simulink library "tpm"  (R2021b)
settings: Solver=VariableStepAuto  StartTime=0.0  StopTime=10.0  RelTol=1e-3
undefined symbols (not defined in the file or in its folder): ENUM_AN_LF, ENUM_AN_LR, ENUM_AN_RF, ENUM_AN_RR, ENUM_POWERSTA_OFF, ENUM_POWERSTA_OFFA, ENUM_POWERSTA_OFFC, ENUM_POWERSTA_ON, ENUM_POWERSTA_READY, ENUM_POWERSTA_STANDBY, ENUM_PWRSTASW_OFF, ENUM_PWRSTASW_OFFA, ENUM_PWRSTASW_OFFCHVCHRG, ENUM_PWRSTASW_STANDBY, KTPM_Delay_raw8, KTPM_WhlRotDir_enum_ovrdflg, KTPM_WhlRotDir_enum_ovrdval, TRUE, ZERO_FLOAT, ZERO_INT
libraries: simulink x58, hcu_lib x25, $bdroot x18
(part 1 of 8)
settings Model: Creator=FVT22063  LastModifiedBy=FVT22063

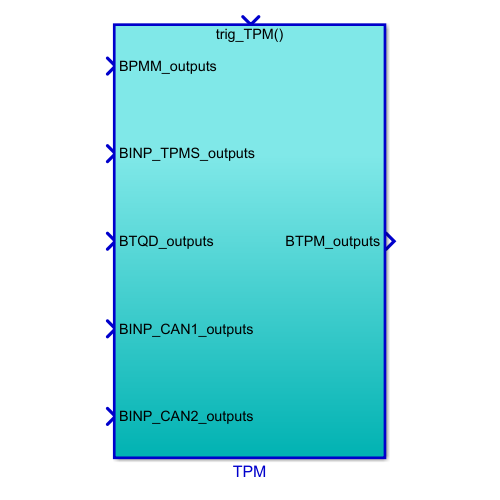
[thumbnail: Simulink's stored preview of the top-level diagram]
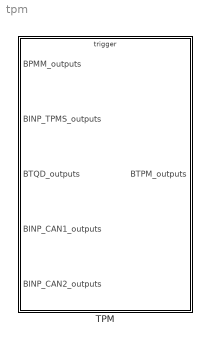
== system tpm ==
  TPM : Subsystem  TreatAsAtomicUnit=on
      settings: RTWSystemCode=Nonreusable function  RTWFcnNameOpts=Use subsystem name  RTWFileNameOpts=Use subsystem name

== system tpm/TPM ==
  note: VINP
  BPMM_outputs : Inport  OutDataTypeStr=Bus: BPMM_outputs
  BINP_TPMS_outputs : Inport  Port=2  OutDataTypeStr=Bus: BINP_TPMS_outputs
  BTQD_outputs : Inport  Port=3  OutDataTypeStr=Bus: BTQD_outputs
  BINP_CAN1_outputs : Inport  Port=4  OutDataTypeStr=Bus: BINP_CAN1_outputs
  BINP_CAN2_outputs : Inport  Port=5  OutDataTypeStr=Bus: BINP_CAN2_outputs
  trig_TPM : TriggerPort  TriggerType=function-call  VariantControl=(inherit)
  Bus Creator : BusCreator  Inputs=108  OutDataTypeStr=Bus: BTPM_outputs  NonVirtualBus=on
  Bus Selector : BusSelector  OutputSignals=VPMM_PowerSta_enum
  Bus Selector1 : BusSelector  OutputSignals=VINP_TPMSDataIn_flg,VINP_TPMSID_raw,VINP_TPMSPressure_raw,VINP_TPMSTemp_raw,VINP_TPMSFAT_flg,VINP_TPMSBattLow_flg,VINP_TPMSStorge_flg,VINP_LFID_raw,VINP_RFID_raw,VINP_LRID_raw,VINP_RRID_raw,VINP_ChkStorge_flg,VINP_ChkLFID_raw,VINP_ChkRFID_raw,VINP_ChkLRID_raw,VINP_ChkRRID_raw,VINP_FlashLFSensorFail_flg,VINP_FlashRFSensorFail_flg,VINP_FlashLRSensorFail_flg,VINP_FlashRRSensorFail_flg,VINP_FlashLFWheelPSW_raw8,VINP_FlashRFWheelPSW_raw8,VINP_FlashLRWheelPSW_raw8,VINP_FlashRRWheelPSW_raw8,VINP_FlashLFPindi_enum,VINP_FlashRFPindi_enum,VINP_FlashLRPindi_enum,VINP_FlashRRPindi_enum,VINP_FlashLFP20_raw8,VINP_FlashRFP20_raw8,VINP_FlashLRP20_raw8,VINP_FlashRRP20_raw8,VINP_FlashLFWheelPress_raw8,VINP_FlashRFWheelPress_raw8,VINP_FlashLRWheelPress_raw8,VINP_FlashRRWheelPress_raw8,VINP_FlashLFWheelTemp_C,VINP_FlashRFWheelTemp_C,VINP_FlashLRWheelTemp_C,VINP_FlashRRWheelTemp_C,VINP_FlashunlearnSfali_flg,VINP_S1ID_raw,VINP_S2ID_raw,VINP_S3ID_raw,VINP_S4ID_raw,VINP_Prepresstemptrust_flg
  Bus Selector2 : BusSelector  OutputSignals=VTQD_GearActualPosn_enum
  Bus Selector3 : BusSelector  OutputSignals=VINP_FASpeed_kph
  Bus Selector4 : BusSelector  OutputSignals=VINP_TPMSResButt_flg,VINP_TPMSCaliButt_flg,VINP_CANMsgValidIVI2_flg
  Data Type Conversion{,1..7} (8 alike) : DataTypeConversion  OutDataTypeStr=uint8
  Data Type Conversion{8..11} (4 alike) : DataTypeConversion  OutDataTypeStr=boolean
  Ground{,1..11} (12 alike) : Ground
  TPMS : Subsystem
  BTPM_outputs : Outport  OutDataTypeStr=Bus: BTPM_outputs
  wires:
  BPMM_outputs/1 -> Bus Selector/1
  BINP_TPMS_outputs/1 -> Bus Selector1/1
  BTQD_outputs/1 -> Bus Selector2/1
  BINP_CAN1_outputs/1 -> Bus Selector3/1
  BINP_CAN2_outputs/1 -> Bus Selector4/1
  Bus Creator/1 -> BTPM_outputs/1  "BTPM_outputs"
  Bus Selector/1 -> TPMS/1(VPMM_PowerSta_enum)  "<VPMM_PowerSta_enum>"
  Bus Selector1/1 -> TPMS/2(VINP_DATAin_flg)  "<VINP_TPMSDataIn_flg>"
  Bus Selector1/2 -> TPMS/3(VINP_IDin_raw32)  "<VINP_TPMSID_raw>"
  Bus Selector1/3 -> TPMS/4(VINP_Pin_raw8)  "<VINP_TPMSPressure_raw>"
  Bus Selector1/4 -> TPMS/5(VINP_Tin_raw8)  "<VINP_TPMSTemp_raw>"
  Bus Selector1/5 -> TPMS/6(VINP_FAT_flg)  "<VINP_TPMSFAT_flg>"
  Bus Selector1/6 -> TPMS/7(VINP_BatteryLow_flg)  "<VINP_TPMSBattLow_flg>"
  Bus Selector1/7 -> TPMS/8(VINP_TPMSStorge_flg)  "<VINP_TPMSStorge_flg>"
  Bus Selector1/8 -> TPMS/9(VINP_LFID_raw)  "<VINP_LFID_raw>"
  Bus Selector1/9 -> TPMS/10(VINP_RFID_raw)  "<VINP_RFID_raw>"
  Bus Selector1/10 -> TPMS/11(VINP_LRID_raw)  "<VINP_LRID_raw>"
  Bus Selector1/11 -> TPMS/12(VINP_RRID_raw)  "<VINP_RRID_raw>"
  Bus Selector1/12 -> TPMS/13(VINP_ChkStorge_flg)  "<VINP_ChkStorge_flg>"
  Bus Selector1/13 -> TPMS/14(VINP_ChkLFID_raw)  "<VINP_ChkLFID_raw>"
  Bus Selector1/14 -> TPMS/15(VINP_ChkRFID_raw)  "<VINP_ChkRFID_raw>"
  Bus Selector1/15 -> TPMS/16(VINP_ChkLRID_raw)  "<VINP_ChkLRID_raw>"
  Bus Selector1/16 -> TPMS/17(VINP_ChkRRID_raw)  "<VINP_ChkRRID_raw>"
  TPMS/14(VTPM_RFSensorFail_flg) -> Bus Creator/14
  TPMS/13(VTPM_LFSensorFail_flg) -> Bus Creator/13
  TPMS/15(VTPM_LRSensorFail_flg) -> Bus Creator/15
  TPMS/12(VTPM_RRWheelTemp_C) -> Bus Creator/12
  TPMS/16(VTPM_RRSensorFail_flg) -> Bus Creator/16
  TPMS/11("VTPM_LRWheelTemp_C ") -> Bus Creator/11
  TPMS/17(VTPM_LFWheelDebug_flg) -> Bus Creator/17
  TPMS/10("VTPM_RFWheelTemp_C ") -> Bus Creator/10
  TPMS/18(VTPM_LRWheelDebug_flg) -> Bus Creator/18
  TPMS/9("VTPM_LFWheelTemp_C ") -> Bus Creator/9
  TPMS/19(VTPM_RFWheelDebug_flg) -> Bus Creator/19
  TPMS/8(VTPM_RRWheelPress_raw8) -> Bus Creator/8
  TPMS/20(VTPM_RRWheelDebug_flg) -> Bus Creator/20
  TPMS/7(VTPM_LRWheelPress_raw8) -> Bus Creator/7
  TPMS/21(VTPM_TPMSResButtAllow_flg) -> Bus Creator/21
  TPMS/6(VTPM_RFWheelPress_raw8) -> Bus Creator/6
  TPMS/22(VTPM_TPMSCaliButtAllow_flg) -> Bus Creator/22
  TPMS/5(VTPM_LFWheelPress_raw8) -> Bus Creator/5
  TPMS/23(VTPM_LFPressIndi_enum) -> Bus Creator/23
  TPMS/4("VTPM_RRBatWarn_flg ") -> Bus Creator/4
  TPMS/24(VTPM_RFPressIndi_enum) -> Bus Creator/24
  TPMS/3("VTPM_LRBatWarn_flg ") -> Bus Creator/3
  TPMS/25(VTPM_LRPressIndi_enum) -> Bus Creator/25
  TPMS/2("VTPM_RFBatWarn_flg ") -> Bus Creator/2
  TPMS/26(VTPM_RRPressIndi_enum) -> Bus Creator/26
  TPMS/1("VTPM_LFBatWarn_flg ") -> Bus Creator/1
  TPMS/27("VTPM_TPMSWarnIndi_enum ") -> Bus Creator/27
  TPMS/28(VTPM_LFWheelTmpIndi_flg) -> Bus Creator/28
  TPMS/29(VTPM_RFWheelTmpIndi_flg) -> Bus Creator/29
  TPMS/30(VTPM_LRWheelTmpIndi_flg) -> Bus Creator/30
  TPMS/31(VTPM_RRWheelTmpIndi_flg) -> Bus Creator/31
  TPMS/32(VTPM_LFWheelPSW_raw8) -> Bus Creator/32
  TPMS/33(VTPM_LRWheelPSW_raw8) -> Bus Creator/33
  TPMS/34(VTPM_RFWheelPSW_raw8) -> Bus Creator/34
  TPMS/35(VTPM_RRWheelPSW_raw8) -> Bus Creator/35
  TPMS/36(VTPM_LFS1_cnt) -> Bus Creator/36
  TPMS/37(VTPM_RFS1_cnt) -> Bus Creator/37
  TPMS/38(VTPM_RRS1_cnt) -> Bus Creator/38
  TPMS/39(VTPM_LRS1_cnt) -> Bus Creator/39
  TPMS/40(VTPM_LFS2_cnt) -> Bus Creator/40
  TPMS/41(VTPM_RFS2_cnt) -> Bus Creator/41
  TPMS/42(VTPM_RRS2_cnt) -> Bus Creator/42
  TPMS/43(VTPM_LRS2_cnt) -> Bus Creator/43
  TPMS/44(VTPM_LFS3_cnt) -> Bus Creator/44
  TPMS/45(VTPM_RFS3_cnt) -> Bus Creator/45
  TPMS/46(VTPM_RRS3_cnt) -> Bus Creator/46
  TPMS/47(VTPM_LRS3_cnt) -> Bus Creator/47
  TPMS/48(VTPM_LFS4_cnt) -> Bus Creator/48
  TPMS/49(VTPM_RFS4_cnt) -> Bus Creator/49
  TPMS/50(VTPM_RRS4_cnt) -> Bus Creator/50
  TPMS/51(VTPM_LRS4_cnt) -> Bus Creator/51
  TPMS/52(VTPM_CWheelTips_enum) -> Bus Creator/52
  TPMS/53(VTPM_AutoLTips_enum) -> Bus Creator/53
  TPMS/54(VTPM_LFSensorMode_flg) -> Bus Creator/54
  TPMS/55(VTPM_RFSensorMode_flg) -> Bus Creator/55
  TPMS/56(VTPM_LRSensorMode_flg) -> Bus Creator/56
  TPMS/57(VTPM_RRSensorMode_flg) -> Bus Creator/57
  TPMS/58(VTPM_S1ID_raw32) -> Bus Creator/58
  TPMS/59(VTPM_S2ID_raw32) -> Bus Creator/59
  TPMS/60(VTPM_S3ID_raw32) -> Bus Creator/60
  TPMS/61(VTPM_S4ID_raw32) -> Bus Creator/61
  TPMS/62(VTPM_S1L_enum) -> Bus Creator/62
  TPMS/63(VTPM_S2L_enum) -> Bus Creator/63
  TPMS/64(VTPM_S3L_enum) -> Bus Creator/64
  TPMS/65(VTPM_S4L_enum) -> Bus Creator/65
  TPMS/66(VTPM_ALFin_flg) -> Bus Creator/66
  TPMS/67(VTPM_IDLOCK_flg) -> Bus Creator/67
  TPMS/68(VTPM_LFP20_raw8) -> Bus Creator/68
  TPMS/69(VTPM_RFP20_raw8) -> Bus Creator/69
  TPMS/70(VTPM_LRP20_raw8) -> Bus Creator/70
  TPMS/71(VTPM_RRP20_raw8) -> Bus Creator/71
  TPMS/72(VTPM_FAT_flg) -> Bus Creator/72
  TPMS/73(VTPM_IDin_raw32) -> Bus Creator/73
  TPMS/74(VTPM_S1WheelDebugALTU_pct) -> Bus Creator/74
  TPMS/75(VTPM_S2WheelDebugALTU_pct) -> Bus Creator/75
  TPMS/76(VTPM_S3WheelDebugALTU_pct) -> Bus Creator/76
  TPMS/77(VTPM_S4WheelDebugALTU_pct) -> Bus Creator/77
  TPMS/78(VTPM_ID1messageALTU_raw8) -> Bus Creator/78
  TPMS/79(VTPM_ID2messageALTU_raw8) -> Bus Creator/79
  TPMS/80(VTPM_ID3messageALTU_raw8) -> Bus Creator/80
  TPMS/81(VTPM_ID4messageALTU_raw8) -> Bus Creator/81
  TPMS/82(VTPM_Chkfin_flg) -> Bus Creator/82
  TPMS/83(VTPM_SetIDLoc_flg) -> Bus Creator/83
  TPMS/84(VTPM_TPMSStorge_flg) -> Bus Creator/84
  TPMS/85(VTPM_ChkStorge_flg) -> Bus Creator/85
  TPMS/86(VTPM_TPMSResButt_flg) -> Bus Creator/86
  TPMS/87(VTPM_LFPindi_enum) -> Bus Creator/87
  TPMS/88(VTPM_RFPind_enum) -> Bus Creator/88
  TPMS/89(VTPM_LRPindi_enum) -> Bus Creator/89
  TPMS/90(VTPM_RRPindi_enum) -> Bus Creator/90
  TPMS/91(VTPM_WriteChkLFID_raw) -> Bus Creator/91
  TPMS/92(VTPM_WriteChkRFID_raw) -> Bus Creator/92
  TPMS/93(VTPM_WriteChkLRID_raw) -> Bus Creator/93
  TPMS/94(VTPM_WriteChkRRID_raw) -> Bus Creator/94
  TPMS/95(VTPM_WriteChkfinLFID_raw) -> Bus Creator/95
  TPMS/96(VTPM_WriteChkfinRFID_raw) -> Bus Creator/96
  TPMS/97(VTPM_WriteChkfinLRID_raw) -> Bus Creator/97
  TPMS/98(VTPM_WriteChkfinRRID_raw) -> Bus Creator/98
  TPMS/99(VTPM_Flashchkdatavalid_enum) -> Bus Creator/99
  TPMS/100(VTPM_Flashdatavalid_enum) -> Bus Creator/100
  TPMS/101(VTPM_unlearnSfali_flg) -> Bus Creator/101
  Bus Selector1/17 -> TPMS/18(VINP_FlashLFSensorFail_flg)  "<VINP_FlashLFSensorFail_flg>"
  Bus Selector1/18 -> TPMS/19(VINP_FlashRFSensorFail_flg)  "<VINP_FlashRFSensorFail_flg>"
  Bus Selector1/19 -> TPMS/20(VINP_FlashLRSensorFail_flg)  "<VINP_FlashLRSensorFail_flg>"
  Bus Selector1/20 -> TPMS/21(VINP_FlashRRSensorFail_flg)  "<VINP_FlashRRSensorFail_flg>"
  Bus Selector1/21 -> TPMS/22(VINP_FlashLFWheelPSW_raw8)  "<VINP_FlashLFWheelPSW_raw8>"
  Bus Selector1/22 -> TPMS/23(VINP_FlashRFWheelPSW_raw8)  "<VINP_FlashRFWheelPSW_raw8>"
  Bus Selector1/23 -> TPMS/24(VINP_FlashLRWheelPSW_raw8)  "<VINP_FlashLRWheelPSW_raw8>"
  Bus Selector1/24 -> TPMS/25(VINP_FlashRRWheelPSW_raw8)  "<VINP_FlashRRWheelPSW_raw8>"
  Bus Selector1/25 -> TPMS/26(VINP_FlashLFPindi_enum)  "<VINP_FlashLFPindi_enum>"
  Bus Selector1/26 -> TPMS/27(VINP_FlashRFPindi_enum)  "<VINP_FlashRFPindi_enum>"
  Bus Selector1/27 -> TPMS/28(VINP_FlashLRPindi_enum)  "<VINP_FlashLRPindi_enum>"
  Bus Selector1/28 -> TPMS/29(VINP_FlashRRPindi_enum)  "<VINP_FlashRRPindi_enum>"
  Bus Selector1/29 -> TPMS/30(VINP_FlashLFP20_raw8)  "<VINP_FlashLFP20_raw8>"
  Bus Selector1/30 -> TPMS/31(VINP_FlashRFP20_raw8)  "<VINP_FlashRFP20_raw8>"
  Bus Selector1/31 -> TPMS/32(VINP_FlashLRP20_raw8)  "<VINP_FlashLRP20_raw8>"
  Bus Selector1/32 -> TPMS/33(VINP_FlashRRP20_raw8)  "<VINP_FlashRRP20_raw8>"
  Bus Selector1/33 -> TPMS/34(VINP_FlashLFWheelPress_raw8)  "<VINP_FlashLFWheelPress_raw8>"
  Bus Selector1/34 -> TPMS/35(VINP_FlashRFWheelPress_raw8)  "<VINP_FlashRFWheelPress_raw8>"
  Bus Selector1/35 -> TPMS/36(VINP_FlashLRFWheelPress_raw8)  "<VINP_FlashLRWheelPress_raw8>"
  Bus Selector1/36 -> TPMS/37(VINP_FlashRRWheelPress_raw8)  "<VINP_FlashRRWheelPress_raw8>"
  Bus Selector1/37 -> TPMS/38(VINP_FlashLFWheelTemp_C)  "<VINP_FlashLFWheelTemp_C>"
  Bus Selector1/38 -> TPMS/39(VINP_FlashRFWheelTemp_C)  "<VINP_FlashRFWheelTemp_C>"
  Bus Selector1/39 -> TPMS/40(VINP_FlashLRWheelTemp_C)  "<VINP_FlashLRWheelTemp_C>"
  Bus Selector1/40 -> TPMS/41(VINP_FlashRRWheelTemp_C)  "<VINP_FlashRRWheelTemp_C>"
  Bus Selector1/41 -> TPMS/42(VINP_FlashunlearnSfali_flg)  "<VINP_FlashunlearnSfali_flg>"
  Bus Selector4/1 -> TPMS/61(VINP_TPMSResButt_flg)  "<VINP_TPMSResButt_flg>"
  Bus Selector4/2 -> TPMS/62(VINP_TPMSCaliButt_flg)  "<VINP_TPMSCaliButt_flg>"
  Bus Selector4/3 -> TPMS/63(VINP_IVICANValid_flg)  "<VINP_CANMsgValidIVI2_flg>"
  Bus Selector2/1 -> TPMS/64(VTQD_GearActualPosn_enum)  "<VTQD_GearActualPosn_enum>"
  TPMS/102(VTPM_unlearnSfailvalid_enum) -> Bus Creator/102
  TPMS/103(VTPM_Prepresstempvalid_enum) -> Bus Creator/103
  Bus Selector1/42 -> TPMS/43(VINP_S1ID_raw)  "<VINP_S1ID_raw>"
  Bus Selector1/43 -> TPMS/44(VINP_S2ID_raw)  "<VINP_S2ID_raw>"
  Bus Selector1/44 -> TPMS/45(VINP_S3ID_raw)  "<VINP_S3ID_raw>"
  Bus Selector1/45 -> TPMS/46(VINP_S4ID_raw)  "<VINP_S4ID_raw>"
  TPMS/104(VTPM_FlashS1ID_raw) -> Bus Creator/104
  TPMS/105(VTPM_FlashS2ID_raw) -> Bus Creator/105
  TPMS/106(VTPM_FlashS3ID_raw) -> Bus Creator/106
  TPMS/107(VTPM_FlashS4ID_raw) -> Bus Creator/107
  TPMS/108(VTPM_FlashIDvalid_enum) -> Bus Creator/108
  Bus Selector1/46 -> TPMS/47(VINP_Prepresstemptrust_flg)  "<VINP_Prepresstemptrust_flg>"
  Bus Selector3/1 -> TPMS/60(VINP_VehSpeed_kph)  "<VINP_FASpeed_kph>"
  Ground/1 -> Data Type Conversion/1
  Ground1/1 -> Data Type Conversion1/1
  Ground2/1 -> Data Type Conversion2/1
  Ground3/1 -> Data Type Conversion3/1
  Ground4/1 -> Data Type Conversion8/1
  Ground5/1 -> Data Type Conversion9/1
  Ground6/1 -> Data Type Conversion10/1
  Ground7/1 -> Data Type Conversion11/1
  Ground8/1 -> Data Type Conversion4/1
  Ground9/1 -> Data Type Conversion5/1
  Ground10/1 -> Data Type Conversion6/1
  Ground11/1 -> Data Type Conversion7/1
  Data Type Conversion/1 -> TPMS/48(VINP_LFPulseCount_cnt)
  Data Type Conversion1/1 -> TPMS/49(VINP_RFPulseCount_cnt)
  Data Type Conversion2/1 -> TPMS/50(VINP_LRPulseCount_cnt)
  Data Type Conversion3/1 -> TPMS/51(VINP_RRPulseCount_cnt)
  Data Type Conversion4/1 -> TPMS/56(VINP_LFWhlRotDir_enum)
  Data Type Conversion5/1 -> TPMS/57(VINP_RFWhlRotDir_enum)
  Data Type Conversion6/1 -> TPMS/58(VINP_LRWhlRotDir_enum)
  Data Type Conversion7/1 -> TPMS/59(VINP_RRWhlRotDir_enum)
  Data Type Conversion8/1 -> TPMS/52(VINP_LFPulseCountV_flg)
  Data Type Conversion9/1 -> TPMS/53(VINP_RFPulseCountV_flg)
  Data Type Conversion10/1 -> TPMS/54(VINP_LRPulseCountV_flg)
  Data Type Conversion11/1 -> TPMS/55(VINP_RRPulseCountV_flg)

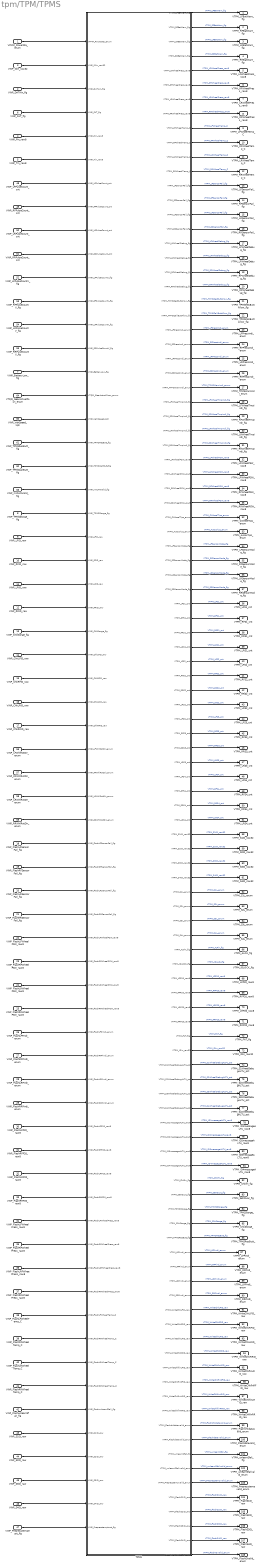
== system tpm/TPM/TPMS ==
  VPMM_PowerSta_enum : Inport
  VINP_DATAin_flg : Inport  Port=2
  VINP_IDin_raw32 : Inport  Port=3
  VINP_Pin_raw8 : Inport  Port=4
  VINP_Tin_raw8 : Inport  Port=5
  VINP_FAT_flg : Inport  Port=6
  VINP_BatteryLow_flg : Inport  Port=7
  VINP_TPMSStorge_flg : Inport  Port=8
  VINP_LFID_raw : Inport  Port=9
  VINP_RFID_raw : Inport  Port=10
  VINP_LRID_raw : Inport  Port=11
  VINP_RRID_raw : Inport  Port=12
  VINP_ChkStorge_flg : Inport  Port=13
  VINP_ChkLFID_raw : Inport  Port=14
  VINP_ChkRFID_raw : Inport  Port=15
  VINP_ChkLRID_raw : Inport  Port=16
  VINP_ChkRRID_raw : Inport  Port=17
  VINP_FlashLFSensorFail_flg : Inport  Port=18
  VINP_FlashRFSensorFail_flg : Inport  Port=19
  VINP_FlashLRSensorFail_flg : Inport  Port=20
  VINP_FlashRRSensorFail_flg : Inport  Port=21
  VINP_FlashLFWheelPSW_raw8 : Inport  Port=22
  VINP_FlashRFWheelPSW_raw8 : Inport  Port=23
  VINP_FlashLRWheelPSW_raw8 : Inport  Port=24
  VINP_FlashRRWheelPSW_raw8 : Inport  Port=25
  VINP_FlashLFPindi_enum : Inport  Port=26
  VINP_FlashRFPindi_enum : Inport  Port=27
  VINP_FlashLRPindi_enum : Inport  Port=28
  VINP_FlashRRPindi_enum : Inport  Port=29
  VINP_FlashLFP20_raw8 : Inport  Port=30
  VINP_FlashRFP20_raw8 : Inport  Port=31
  VINP_FlashLRP20_raw8 : Inport  Port=32
  VINP_FlashRRP20_raw8 : Inport  Port=33
  VINP_FlashLFWheelPress_raw8 : Inport  Port=34
  VINP_FlashRFWheelPress_raw8 : Inport  Port=35
  VINP_FlashLRFWheelPress_raw8 : Inport  Port=36
  VINP_FlashRRWheelPress_raw8 : Inport  Port=37
  VINP_FlashLFWheelTemp_C : Inport  Port=38
  VINP_FlashRFWheelTemp_C : Inport  Port=39
  VINP_FlashLRWheelTemp_C : Inport  Port=40
  VINP_FlashRRWheelTemp_C : Inport  Port=41
  VINP_FlashunlearnSfali_flg : Inport  Port=42
  VINP_S1ID_raw : Inport  Port=43
  VINP_S2ID_raw : Inport  Port=44
  VINP_S3ID_raw : Inport  Port=45
  VINP_S4ID_raw : Inport  Port=46
  VINP_Prepresstemptrust_flg : Inport  Port=47
  VINP_LFPulseCount_cnt : Inport  Port=48
  VINP_RFPulseCount_cnt : Inport  Port=49
  VINP_LRPulseCount_cnt : Inport  Port=50
  VINP_RRPulseCount_cnt : Inport  Port=51
  VINP_LFPulseCountV_flg : Inport  Port=52
  VINP_RFPulseCountV_flg : Inport  Port=53
  VINP_LRPulseCountV_flg : Inport  Port=54
  VINP_RRPulseCountV_flg : Inport  Port=55
  VINP_LFWhlRotDir_enum : Inport  Port=56
  VINP_RFWhlRotDir_enum : Inport  Port=57
  VINP_LRWhlRotDir_enum : Inport  Port=58
  VINP_RRWhlRotDir_enum : Inport  Port=59
  VINP_VehSpeed_kph : Inport  Port=60
  VINP_TPMSResButt_flg : Inport  Port=61
  VINP_TPMSCaliButt_flg : Inport  Port=62
  VINP_IVICANValid_flg : Inport  Port=63
  VTQD_GearActualPosn_enum : Inport  Port=64
  TPMS : Subsystem
  "VTPM_LFBatWarn_flg " : Outport
  "VTPM_RFBatWarn_flg " : Outport  Port=2
  "VTPM_LRBatWarn_flg " : Outport  Port=3
  "VTPM_RRBatWarn_flg " : Outport  Port=4
  VTPM_LFWheelPress_raw8 : Outport  Port=5
  VTPM_RFWheelPress_raw8 : Outport  Port=6
  VTPM_LRWheelPress_raw8 : Outport  Port=7
  VTPM_RRWheelPress_raw8 : Outport  Port=8
  "VTPM_LFWheelTemp_C " : Outport  Port=9
  "VTPM_RFWheelTemp_C " : Outport  Port=10
  "VTPM_LRWheelTemp_C " : Outport  Port=11
  VTPM_RRWheelTemp_C : Outport  Port=12
  VTPM_LFSensorFail_flg : Outport  Port=13
  VTPM_RFSensorFail_flg : Outport  Port=14
  VTPM_LRSensorFail_flg : Outport  Port=15
  VTPM_RRSensorFail_flg : Outport  Port=16
  VTPM_LFWheelDebug_flg : Outport  Port=17
  VTPM_LRWheelDebug_flg : Outport  Port=18
  VTPM_RFWheelDebug_flg : Outport  Port=19
  VTPM_RRWheelDebug_flg : Outport  Port=20
  VTPM_TPMSResButtAllow_flg : Outport  Port=21
  VTPM_TPMSCaliButtAllow_flg : Outport  Port=22
  VTPM_LFPressIndi_enum : Outport  Port=23
  VTPM_RFPressIndi_enum : Outport  Port=24
  VTPM_LRPressIndi_enum : Outport  Port=25
  VTPM_RRPressIndi_enum : Outport  Port=26
  "VTPM_TPMSWarnIndi_enum " : Outport  Port=27
  VTPM_LFWheelTmpIndi_flg : Outport  Port=28
  VTPM_RFWheelTmpIndi_flg : Outport  Port=29
  VTPM_LRWheelTmpIndi_flg : Outport  Port=30
  VTPM_RRWheelTmpIndi_flg : Outport  Port=31
  VTPM_LFWheelPSW_raw8 : Outport  Port=32
  VTPM_LRWheelPSW_raw8 : Outport  Port=33
  VTPM_RFWheelPSW_raw8 : Outport  Port=34
  VTPM_RRWheelPSW_raw8 : Outport  Port=35
  VTPM_LFS1_cnt : Outport  Port=36
  VTPM_RFS1_cnt : Outport  Port=37
  VTPM_RRS1_cnt : Outport  Port=38
  VTPM_LRS1_cnt : Outport  Port=39
  VTPM_LFS2_cnt : Outport  Port=40
  VTPM_RFS2_cnt : Outport  Port=41
  VTPM_RRS2_cnt : Outport  Port=42
  VTPM_LRS2_cnt : Outport  Port=43
  VTPM_LFS3_cnt : Outport  Port=44
  VTPM_RFS3_cnt : Outport  Port=45
  VTPM_RRS3_cnt : Outport  Port=46
  VTPM_LRS3_cnt : Outport  Port=47
  VTPM_LFS4_cnt : Outport  Port=48
  VTPM_RFS4_cnt : Outport  Port=49
  VTPM_RRS4_cnt : Outport  Port=50
  VTPM_LRS4_cnt : Outport  Port=51
  VTPM_CWheelTips_enum : Outport  Port=52
  VTPM_AutoLTips_enum : Outport  Port=53
  VTPM_LFSensorMode_flg : Outport  Port=54
  VTPM_RFSensorMode_flg : Outport  Port=55
  VTPM_LRSensorMode_flg : Outport  Port=56
  VTPM_RRSensorMode_flg : Outport  Port=57
  VTPM_S1ID_raw32 : Outport  Port=58
  VTPM_S2ID_raw32 : Outport  Port=59
  VTPM_S3ID_raw32 : Outport  Port=60
  VTPM_S4ID_raw32 : Outport  Port=61
  VTPM_S1L_enum : Outport  Port=62
  VTPM_S2L_enum : Outport  Port=63
  VTPM_S3L_enum : Outport  Port=64
  VTPM_S4L_enum : Outport  Port=65
  VTPM_ALFin_flg : Outport  Port=66
  VTPM_IDLOCK_flg : Outport  Port=67
  VTPM_LFP20_raw8 : Outport  Port=68
  VTPM_RFP20_raw8 : Outport  Port=69
  VTPM_LRP20_raw8 : Outport  Port=70
  VTPM_RRP20_raw8 : Outport  Port=71
  VTPM_FAT_flg : Outport  Port=72
  VTPM_IDin_raw32 : Outport  Port=73
  VTPM_S1WheelDebugALTU_pct : Outport  Port=74
  VTPM_S2WheelDebugALTU_pct : Outport  Port=75
  VTPM_S3WheelDebugALTU_pct : Outport  Port=76
  VTPM_S4WheelDebugALTU_pct : Outport  Port=77
  VTPM_ID1messageALTU_raw8 : Outport  Port=78
  VTPM_ID2messageALTU_raw8 : Outport  Port=79
  VTPM_ID3messageALTU_raw8 : Outport  Port=80
  VTPM_ID4messageALTU_raw8 : Outport  Port=81
  VTPM_Chkfin_flg : Outport  Port=82
  VTPM_SetIDLoc_flg : Outport  Port=83
  VTPM_TPMSStorge_flg : Outport  Port=84
  VTPM_ChkStorge_flg : Outport  Port=85
  VTPM_TPMSResButt_flg : Outport  Port=86
  VTPM_LFPindi_enum : Outport  Port=87
  VTPM_RFPind_enum : Outport  Port=88
  VTPM_LRPindi_enum : Outport  Port=89
  VTPM_RRPindi_enum : Outport  Port=90
  VTPM_WriteChkLFID_raw : Outport  Port=91
  VTPM_WriteChkRFID_raw : Outport  Port=92
  VTPM_WriteChkLRID_raw : Outport  Port=93
  VTPM_WriteChkRRID_raw : Outport  Port=94
  VTPM_WriteChkfinLFID_raw : Outport  Port=95
  VTPM_WriteChkfinRFID_raw : Outport  Port=96
  VTPM_WriteChkfinLRID_raw : Outport  Port=97
  VTPM_WriteChkfinRRID_raw : Outport  Port=98
  VTPM_Flashchkdatavalid_enum : Outport  Port=99
  VTPM_Flashdatavalid_enum : Outport  Port=100
  VTPM_unlearnSfali_flg : Outport  Port=101
  VTPM_unlearnSfailvalid_enum : Outport  Port=102
  VTPM_Prepresstempvalid_enum : Outport  Port=103
  VTPM_FlashS1ID_raw : Outport  Port=104
  VTPM_FlashS2ID_raw : Outport  Port=105
  VTPM_FlashS3ID_raw : Outport  Port=106
  VTPM_FlashS4ID_raw : Outport  Port=107
  VTPM_FlashIDvalid_enum : Outport  Port=108
  wires:
  TPMS/87(VTPM_LFPindi_enum) -> VTPM_LFPindi_enum/1  "VTPM_LFPindi_enum"
  TPMS/1("VTPM_LFBatWarn_flg ") -> "VTPM_LFBatWarn_flg "/1  "VTPM_LFBatWarn_flg"
  TPMS/2("VTPM_RFBatWarn_flg ") -> "VTPM_RFBatWarn_flg "/1  "VTPM_RFBatWarn_flg"
  TPMS/3("VTPM_LRBatWarn_flg ") -> "VTPM_LRBatWarn_flg "/1  "VTPM_LRBatWarn_flg"
  TPMS/4("VTPM_RRBatWarn_flg ") -> "VTPM_RRBatWarn_flg "/1  "VTPM_RRBatWarn_flg"
  TPMS/5(VTPM_LFWheelPress_raw8) -> VTPM_LFWheelPress_raw8/1  "VTPM_LFWheelPress_raw8"
  TPMS/6(VTPM_RFWheelPress_raw8) -> VTPM_RFWheelPress_raw8/1  "VTPM_RFWheelPress_raw8"
  TPMS/7(VTPM_LRWheelPress_raw8) -> VTPM_LRWheelPress_raw8/1  "VTPM_LRWheelPress_raw8"
  TPMS/8(VTPM_RRWheelPress_raw8) -> VTPM_RRWheelPress_raw8/1  "VTPM_RRWheelPress_raw8"
  TPMS/9("VTPM_LFWheelTemp_C ") -> "VTPM_LFWheelTemp_C "/1  "VTPM_LFWheelTemp_C"
  TPMS/10("VTPM_RFWheelTemp_C ") -> "VTPM_RFWheelTemp_C "/1  "VTPM_RFWheelTemp_C"
  TPMS/11("VTPM_LRWheelTemp_C ") -> "VTPM_LRWheelTemp_C "/1  "VTPM_LRWheelTemp_C"
  TPMS/12(VTPM_RRWheelTemp_C) -> VTPM_RRWheelTemp_C/1  "VTPM_RRWheelTemp_C"
  TPMS/13(VTPM_LFSensorFail_flg) -> VTPM_LFSensorFail_flg/1  "VTPM_LFSensorFail_flg"
  TPMS/14(VTPM_RFSensorFail_flg) -> VTPM_RFSensorFail_flg/1  "VTPM_RFSensorFail_flg"
  TPMS/15(VTPM_LRSensorFail_flg) -> VTPM_LRSensorFail_flg/1  "VTPM_LRSensorFail_flg"
  TPMS/16(VTPM_RRSensorFail_flg) -> VTPM_RRSensorFail_flg/1  "VTPM_RRSensorFail_flg"
  TPMS/17(VTPM_LFWheelDebug_flg) -> VTPM_LFWheelDebug_flg/1  "VTPM_LFWheelDebug_flg"
  TPMS/18(VTPM_LRWheelDebug_flg) -> VTPM_LRWheelDebug_flg/1  "VTPM_LRWheelDebug_flg"
  TPMS/19(VTPM_RFWheelDebug_flg) -> VTPM_RFWheelDebug_flg/1  "VTPM_RFWheelDebug_flg"
  TPMS/20(VTPM_RRWheelDebug_flg) -> VTPM_RRWheelDebug_flg/1  "VTPM_RRWheelDebug_flg"
  TPMS/21(VTPM_TPMSResButtAllow_flg) -> VTPM_TPMSResButtAllow_flg/1  "VTPM_TPMSResButtAllow_flg"
  TPMS/22(VTPM_TPMSCaliButtAllow_flg) -> VTPM_TPMSCaliButtAllow_flg/1  "VTPM_TPMSCaliButtAllow_flg"
  TPMS/23(VTPM_LFPressIndi_enum) -> VTPM_LFPressIndi_enum/1  "VTPM_LFPressIndi_enum"
  TPMS/24(VTPM_RFPressIndi_enum) -> VTPM_RFPressIndi_enum/1  "VTPM_RFPressIndi_enum"
  TPMS/25(VTPM_LRPressIndi_enum) -> VTPM_LRPressIndi_enum/1  "VTPM_LRPressIndi_enum"
  TPMS/26(VTPM_RRPressIndi_enum) -> VTPM_RRPressIndi_enum/1  "VTPM_RRPressIndi_enum"
  TPMS/27("VTPM_TPMSWarnIndi_enum ") -> "VTPM_TPMSWarnIndi_enum "/1  "VTPM_TPMSWarnIndi_enum"
  TPMS/28(VTPM_LFWheelTmpIndi_flg) -> VTPM_LFWheelTmpIndi_flg/1  "VTPM_LFWheelTmpIndi_flg"
  TPMS/29(VTPM_RFWheelTmpIndi_flg) -> VTPM_RFWheelTmpIndi_flg/1  "VTPM_RFWheelTmpIndi_flg"
  TPMS/30(VTPM_LRWheelTmpIndi_flg) -> VTPM_LRWheelTmpIndi_flg/1  "VTPM_LRWheelTmpIndi_flg"
  TPMS/31(VTPM_RRWheelTmpIndi_flg) -> VTPM_RRWheelTmpIndi_flg/1  "VTPM_RRWheelTmpIndi_flg"
  TPMS/32(VTPM_LFWheelPSW_raw8) -> VTPM_LFWheelPSW_raw8/1  "VTPM_LFWheelPSW_raw8"
  TPMS/33(VTPM_LRWheelPSW_raw8) -> VTPM_LRWheelPSW_raw8/1  "VTPM_LRWheelPSW_raw8"
  TPMS/34(VTPM_RFWheelPSW_raw8) -> VTPM_RFWheelPSW_raw8/1  "VTPM_RFWheelPSW_raw8"
  TPMS/35(VTPM_RRWheelPSW_raw8) -> VTPM_RRWheelPSW_raw8/1  "VTPM_RRWheelPSW_raw8"
  TPMS/36(VTPM_CWheelTips_enum) -> VTPM_CWheelTips_enum/1  "VTPM_CWheelTips_enum"
  TPMS/37(VTPM_AutoLTips_enum) -> VTPM_AutoLTips_enum/1  "VTPM_AutoLTips_enum"
  TPMS/38(VTPM_LFSensorMode_flg) -> VTPM_LFSensorMode_flg/1  "VTPM_LFSensorMode_flg"
  TPMS/39(VTPM_RFSensorMode_flg) -> VTPM_RFSensorMode_flg/1  "VTPM_RFSensorMode_flg"
  TPMS/40(VTPM_LRSensorMode_flg) -> VTPM_LRSensorMode_flg/1  "VTPM_LRSensorMode_flg"
  TPMS/41(VTPM_RRSensorMode_flg) -> VTPM_RRSensorMode_flg/1  "VTPM_RRSensorMode_flg"
  TPMS/42(VTPM_LFS1_cnt) -> VTPM_LFS1_cnt/1  "VTPM_LFS1_cnt"
  TPMS/43(VTPM_RFS1_cnt) -> VTPM_RFS1_cnt/1  "VTPM_RFS1_cnt"
  TPMS/44(VTPM_RRS1_cnt) -> VTPM_RRS1_cnt/1  "VTPM_RRS1_cnt"
  TPMS/45(VTPM_LRS1_cnt) -> VTPM_LRS1_cnt/1  "VTPM_LRS1_cnt"
  TPMS/46(VTPM_LFS2_cnt) -> VTPM_LFS2_cnt/1  "VTPM_LFS2_cnt"
  TPMS/47(VTPM_RFS2_cnt) -> VTPM_RFS2_cnt/1  "VTPM_RFS2_cnt"
  TPMS/48(VTPM_RRS2_cnt) -> VTPM_RRS2_cnt/1  "VTPM_RRS2_cnt"
  TPMS/49(VTPM_LRS2_cnt) -> VTPM_LRS2_cnt/1  "VTPM_LRS2_cnt"
  TPMS/50(VTPM_LFS3_cnt) -> VTPM_LFS3_cnt/1  "VTPM_LFS3_cnt"
  TPMS/51(VTPM_RFS3_cnt) -> VTPM_RFS3_cnt/1  "VTPM_RFS3_cnt"
  TPMS/52(VTPM_RRS3_cnt) -> VTPM_RRS3_cnt/1  "VTPM_RRS3_cnt"
  TPMS/53(VTPM_LRS3_cnt) -> VTPM_LRS3_cnt/1  "VTPM_LRS3_cnt"
  TPMS/54(VTPM_LFS4_cnt) -> VTPM_LFS4_cnt/1  "VTPM_LFS4_cnt"
  TPMS/55(VTPM_RFS4_cnt) -> VTPM_RFS4_cnt/1  "VTPM_RFS4_cnt"
  TPMS/56(VTPM_RRS4_cnt) -> VTPM_RRS4_cnt/1  "VTPM_RRS4_cnt"
  TPMS/57(VTPM_LRS4_cnt) -> VTPM_LRS4_cnt/1  "VTPM_LRS4_cnt"
  TPMS/58(VTPM_S1ID_raw32) -> VTPM_S1ID_raw32/1  "VTPM_S1ID_raw32"
  TPMS/59(VTPM_S2ID_raw32) -> VTPM_S2ID_raw32/1  "VTPM_S2ID_raw32"
  TPMS/60(VTPM_S3ID_raw32) -> VTPM_S3ID_raw32/1  "VTPM_S3ID_raw32"
  TPMS/61(VTPM_S4ID_raw32) -> VTPM_S4ID_raw32/1  "VTPM_S4ID_raw32"
  TPMS/62(VTPM_S1L_enum) -> VTPM_S1L_enum/1  "VTPM_S1L_enum"
  TPMS/63(VTPM_S2L_enum) -> VTPM_S2L_enum/1  "VTPM_S2L_enum"
  TPMS/64(VTPM_S3L_enum) -> VTPM_S3L_enum/1  "VTPM_S3L_enum"
  TPMS/65(VTPM_S4L_enum) -> VTPM_S4L_enum/1  "VTPM_S4L_enum"
  TPMS/66(VTPM_ALFin_flg) -> VTPM_ALFin_flg/1  "VTPM_ALFin_flg"
  TPMS/67(VTPM_IDLOCK_flg) -> VTPM_IDLOCK_flg/1  "VTPM_IDLock_flg"
  TPMS/68(VTPM_LFP20_raw8) -> VTPM_LFP20_raw8/1  "VTPM_LFP20_raw8"
  TPMS/69(VTPM_RFP20_raw8) -> VTPM_RFP20_raw8/1  "VTPM_RFP20_raw8"
  TPMS/70(VTPM_LRP20_raw8) -> VTPM_LRP20_raw8/1  "VTPM_LRP20_raw8"
  TPMS/71(VTPM_RRP20_raw8) -> VTPM_RRP20_raw8/1  "VTPM_RRP20_raw8"
  TPMS/72(VTPM_FAT_flg) -> VTPM_FAT_flg/1  "VTPM_FAT_flg"
  TPMS/73(VTPM_IDin_raw32) -> VTPM_IDin_raw32/1  "VTPM_IDin_raw32"
  TPMS/74(VTPM_S1WheelDebugALTU_pct) -> VTPM_S1WheelDebugALTU_pct/1  "VTPM_S1WheelDebugALTU_pct"
  TPMS/75(VTPM_S2WheelDebugALTU_pct) -> VTPM_S2WheelDebugALTU_pct/1  "VTPM_S2WheelDebugALTU_pct"
  TPMS/76(VTPM_S3WheelDebugALTU_pct) -> VTPM_S3WheelDebugALTU_pct/1  "VTPM_S3WheelDebugALTU_pct"
  TPMS/77(VTPM_S4WheelDebugALTU_pct) -> VTPM_S4WheelDebugALTU_pct/1  "VTPM_S4WheelDebugALTU_pct"
  TPMS/79(VTPM_ID2messageALTU_raw8) -> VTPM_ID2messageALTU_raw8/1  "VTPM_ID2messageALTU_raw8"
  TPMS/80(VTPM_ID3messageALTU_raw8) -> VTPM_ID3messageALTU_raw8/1  "VTPM_ID3messageALTU_raw8"
  TPMS/82(VTPM_Chkfin_flg) -> VTPM_Chkfin_flg/1  "VTPM_Chkfin_flg"
  TPMS/83(VTPM_SetIDLoc_flg) -> VTPM_SetIDLoc_flg/1  "VTPM_SetIDLoc_flg"
  TPMS/84(VTPM_TPMSStorge_flg) -> VTPM_TPMSStorge_flg/1  "VTPM_TPMSStorge_flg"
  TPMS/85(VTPM_ChkStorge_flg) -> VTPM_ChkStorge_flg/1  "VTPM_ChkStorge_flg"
  TPMS/86(VTPM_TPMSResButt_flg) -> VTPM_TPMSResButt_flg/1  "VTPM_TPMSResButt_flg"
  TPMS/88(VTPM_RFPind_enum) -> VTPM_RFPind_enum/1  "VTPM_RFPind_enum"
  TPMS/89(VTPM_LRPindi_enum) -> VTPM_LRPindi_enum/1  "VTPM_LRPindi_enum"
  TPMS/90(VTPM_RRPindi_enum) -> VTPM_RRPindi_enum/1  "VTPM_RRPindi_enum"
  TPMS/91(VTPM_WriteChkLFID_raw) -> VTPM_WriteChkLFID_raw/1  "VTPM_WriteChkLFID_raw"
  TPMS/92(VTPM_WriteChkRFID_raw) -> VTPM_WriteChkRFID_raw/1  "VTPM_WriteChkRFID_raw"
  TPMS/93(VTPM_WriteChkLRID_raw) -> VTPM_WriteChkLRID_raw/1  "VTPM_WriteChkLRID_raw"
  TPMS/95(VTPM_WriteChkfinLFID_raw) -> VTPM_WriteChkfinLFID_raw/1  "VTPM_WriteChkfinLFID_raw"
  TPMS/97(VTPM_WriteChkfinLRID_raw) -> VTPM_WriteChkfinLRID_raw/1  "VTPM_WriteChkfinLRID_raw"
  TPMS/98(VTPM_WriteChkfinRRID_raw) -> VTPM_WriteChkfinRRID_raw/1  "VTPM_WriteChkfinRRID_raw"
  TPMS/99(VTPM_Flashchkdatavalid_enum) -> VTPM_Flashchkdatavalid_enum/1  "VTPM_Flashchkdatavalid_enum"
  TPMS/100(VTPM_Flashdatavalid_enum) -> VTPM_Flashdatavalid_enum/1  "VTPM_Flashdatavalid_enum"
  TPMS/101(VTPM_unlearnSfali_flg) -> VTPM_unlearnSfali_flg/1  "VTPM_unlearnSfali_flg"
  TPMS/102(VTPM_unlearnSfailvalid_enum) -> VTPM_unlearnSfailvalid_enum/1  "VTPM_unlearnSfailvalid_enum"
  TPMS/103(VTPM_Prepresstempvalid_enum) -> VTPM_Prepresstempvalid_enum/1  "VTPM_Prepresstempvalid_enum"
  TPMS/78(VTPM_ID1messageALTU_raw8) -> VTPM_ID1messageALTU_raw8/1  "VTPM_ID1messageALTU_raw8"
  TPMS/81(VTPM_ID4messageALTU_raw8) -> VTPM_ID4messageALTU_raw8/1  "VTPM_ID4messageALTU_raw8"
  TPMS/94(VTPM_WriteChkRRID_raw) -> VTPM_WriteChkRRID_raw/1  "VTPM_WriteChkRRID_raw"
  TPMS/96(VTPM_WriteChkfinRFID_raw) -> VTPM_WriteChkfinRFID_raw/1  "VTPM_WriteChkfinRFID_raw"
  VPMM_PowerSta_enum/1 -> TPMS/1(VPMM_PowerSta_enum)
  VINP_IDin_raw32/1 -> TPMS/2(VINP_IDin_raw32)
  VINP_DATAin_flg/1 -> TPMS/3(VINP_DATAin_flg)
  VINP_FAT_flg/1 -> TPMS/4(VINP_FAT_flg)
  VINP_Pin_raw8/1 -> TPMS/5(VINP_Pin_raw8)
  VINP_Tin_raw8/1 -> TPMS/6(VINP_Tin_raw8)
  VINP_LFPulseCount_cnt/1 -> TPMS/7(VINP_LFPulseCount_cnt)
  VINP_RFPulseCount_cnt/1 -> TPMS/8(VINP_RFPulseCount_cnt)
  VINP_LRPulseCount_cnt/1 -> TPMS/9(VINP_LRPulseCount_cnt)
  VINP_RRPulseCount_cnt/1 -> TPMS/10(VINP_RRPulseCount_cnt)
  VINP_LFPulseCountV_flg/1 -> TPMS/11(VINP_LFPulseCountV_flg)
  VINP_RFPulseCountV_flg/1 -> TPMS/12(VINP_RFPulseCountV_flg)
  VINP_LRPulseCountV_flg/1 -> TPMS/13(VINP_LRPulseCountV_flg)
  VINP_RRPulseCountV_flg/1 -> TPMS/14(VINP_RRPulseCountV_flg)
  VINP_BatteryLow_flg/1 -> TPMS/15(VINP_BatteryLow_flg)
  VTQD_GearActualPosn_enum/1 -> TPMS/16(VTQD_GearActualPosn_enum)
  VINP_VehSpeed_kph/1 -> TPMS/17(VINP_VehSpeed_kph)
  VINP_TPMSResButt_flg/1 -> TPMS/18(VINP_TPMSResButt_flg)
  VINP_TPMSCaliButt_flg/1 -> TPMS/19(VINP_TPMSCaliButt_flg)
  VINP_IVICANValid_flg/1 -> TPMS/20(VINP_IVICANValid_flg)
  VINP_TPMSStorge_flg/1 -> TPMS/21(VINP_TPMSStorge_flg)
  VINP_LFID_raw/1 -> TPMS/22(VINP_LFID_raw)
  VINP_RFID_raw/1 -> TPMS/23(VINP_RFID_raw)
  VINP_LRID_raw/1 -> TPMS/24(VINP_LRID_raw)
  VINP_RRID_raw/1 -> TPMS/25(VINP_RRID_raw)
  VINP_ChkStorge_flg/1 -> TPMS/26(VINP_ChkStorge_flg)
  VINP_ChkLFID_raw/1 -> TPMS/27(VINP_ChkLFID_raw)
  VINP_ChkRFID_raw/1 -> TPMS/28(VINP_ChkRFID_raw)
  VINP_ChkLRID_raw/1 -> TPMS/29(VINP_ChkLRID_raw)
  VINP_ChkRRID_raw/1 -> TPMS/30(VINP_ChkRRID_raw)
  VINP_LFWhlRotDir_enum/1 -> TPMS/31(VINP_LFWhlRotDir_enum)
  VINP_RFWhlRotDir_enum/1 -> TPMS/32(VINP_RFWhlRotDir_enum)
  VINP_LRWhlRotDir_enum/1 -> TPMS/33(VINP_LRWhlRotDir_enum)
  VINP_RRWhlRotDir_enum/1 -> TPMS/34(VINP_RRWhlRotDir_enum)
  VINP_FlashLFSensorFail_flg/1 -> TPMS/35(VINP_FlashLFSensorFail_flg)
  VINP_FlashRFSensorFail_flg/1 -> TPMS/36(VINP_FlashRFSensorFail_flg)
  VINP_FlashLRSensorFail_flg/1 -> TPMS/37(VINP_FlashLRSensorFail_flg)
  VINP_FlashRRSensorFail_flg/1 -> TPMS/38(VINP_FlashRRSensorFail_flg)
  VINP_FlashLFWheelPSW_raw8/1 -> TPMS/39(VINP_FlashLFWheelPSW_raw8)
  VINP_FlashRFWheelPSW_raw8/1 -> TPMS/40(VINP_FlashRFWheelPSW_raw8)
  VINP_FlashLRWheelPSW_raw8/1 -> TPMS/41(VINP_FlashLRWheelPSW_raw8)
  VINP_FlashRRWheelPSW_raw8/1 -> TPMS/42(VINP_FlashRRWheelPSW_raw8)
  VINP_FlashLFPindi_enum/1 -> TPMS/43(VINP_FlashLFPindi_enum)
  VINP_FlashRFPindi_enum/1 -> TPMS/44(VINP_FlashRFPindi_enum)
  VINP_FlashLRPindi_enum/1 -> TPMS/45(VINP_FlashLRPindi_enum)
  VINP_FlashRRPindi_enum/1 -> TPMS/46(VINP_FlashRRPindi_enum)
  VINP_FlashLFP20_raw8/1 -> TPMS/47(VINP_FlashLFP20_raw8)
  VINP_FlashRFP20_raw8/1 -> TPMS/48(VINP_FlashRFP20_raw8)
  VINP_FlashLRP20_raw8/1 -> TPMS/49(VINP_FlashLRP20_raw8)
  VINP_FlashRRP20_raw8/1 -> TPMS/50(VINP_FlashRRP20_raw8)
  VINP_FlashLFWheelPress_raw8/1 -> TPMS/51(VINP_FlashLFWheelPress_raw8)
  VINP_FlashRFWheelPress_raw8/1 -> TPMS/52(VINP_FlashRFWheelPress_raw8)
  VINP_FlashLRFWheelPress_raw8/1 -> TPMS/53(VINP_FlashLRFWheelPress_raw8)
  VINP_FlashRRWheelPress_raw8/1 -> TPMS/54(VINP_FlashRRWheelPress_raw8)
  VINP_FlashLFWheelTemp_C/1 -> TPMS/55(VINP_FlashLFWheelTemp_C)
  VINP_FlashRFWheelTemp_C/1 -> TPMS/56(VINP_FlashRFWheelTemp_C)
  VINP_FlashLRWheelTemp_C/1 -> TPMS/57(VINP_FlashLRWheelTemp_C)
  VINP_FlashRRWheelTemp_C/1 -> TPMS/58(VINP_FlashRRWheelTemp_C)
  VINP_FlashunlearnSfali_flg/1 -> TPMS/59(VINP_FlashunlearnSfali_flg)
  TPMS/104(VTPM_FlashS1ID_raw) -> VTPM_FlashS1ID_raw/1  "VTPM_FlashS1ID_raw"
  TPMS/105(VTPM_FlashS2ID_raw) -> VTPM_FlashS2ID_raw/1  "VTPM_FlashS2ID_raw"
  TPMS/106(VTPM_FlashS3ID_raw) -> VTPM_FlashS3ID_raw/1  "VTPM_FlashS3ID_raw"
  TPMS/107(VTPM_FlashS4ID_raw) -> VTPM_FlashS4ID_raw/1  "VTPM_FlashS4ID_raw"
  TPMS/108(VTPM_FlashIDvalid_enum) -> VTPM_FlashIDvalid_enum/1  "VTPM_FlashIDvalid_enum"
  VINP_S2ID_raw/1 -> TPMS/61(VINP_S2ID_raw)
  VINP_S4ID_raw/1 -> TPMS/63(VINP_S4ID_raw)
  VINP_S3ID_raw/1 -> TPMS/62(VINP_S3ID_raw)
  VINP_S1ID_raw/1 -> TPMS/60(VINP_S1ID_raw)
  VINP_Prepresstemptrust_flg/1 -> TPMS/64(VINP_Prepresstemptrust_flg)
